simulink model "Practica_sincronica"  (R2021a)
settings: Solver=ode23tb  StartTime=0.0  StopTime=10  MaxStep=500e-6  RelTol=1e-4  EnableMultiTasking=on
libraries: fl_lib x2, spsRMSLib x2, spsThreePhaseVIMeasurementLib x2, nesl_utility x2, spsThreePhaseProgrammableVoltageSourceLib x1, spsThreePhaseSeriesRLCLoadLib x1, spsGroundLib x1, spsPowerLib x1, spsSynchronousMachinepuFundamentalLib x1, spsThreePhaseBreakerLib x1, spspowerguiLib x1
settings Model: ExtModeAutoUpdateStatusClock=off  Creator=MathWorks  LastModifiedBy=ontib
settings SolverCC: ZeroCrossAlgorithm=Adaptive  AlgebraicLoopSolver=TrustRegion
settings DataIOCC: LimitDataPoints=on  SaveFormat=Array  SignalLoggingSaveFormat=ModelDataLogs  ReturnWorkspaceOutputs=off
settings OptimizationCC: ExpressionDepthLimit=2147483647  InitFltsAndDblsToZero=on  EfficientMapNaN2IntZero=off  LifeSpan=inf
settings DebuggingCC: UnderspecifiedInitializationDetection=Classic  MergeDetectMultiDrivingBlocksExec=none  CheckExecutionContextPreStartOutputMsg=on  SignalResolutionControl=TryResolveAllWithWarning  SolverPrmCheckMsg=warning  MultiTaskDSMMsg=warning  MultiTaskCondExecSysMsg=none  SigSpecEnsureSampleTimeMsg=none  FcnCallInpInsideContextMsg=warning  StateNameClashWarn=warning  SFUnexpectedBacktrackingDiag=warning  SFNoUnconditionalDefaultTransitionDiag=warning  SFExecutionAtInitializationDiag=none  SFMachineParentedDataDiag=warning  ArithmeticOperatorsInVariantConditions=warning
settings HardwareCC: ProdBitPerPointer=32  ProdBitPerSizeT=32  ProdBitPerPtrDiffT=32  ProdLargestAtomicFloat=None  ProdIntDivRoundTo=Undefined  ProdEndianess=Unspecified  ProdWordSize=32  ProdHWDeviceType=32-bit Generic
settings ModelReferenceCC: PropagateSignalLabelsOutOfModel=off
settings SFSimCC: SimUseLocalCustomCode=off  CustomCodeUndefinedFunction=UseInterfaceOnly
settings RTWCC: RTWUseLocalCustomCode=off
settings CodeAppCC: StateflowObjectComments=on
settings GRTTargetCC: TargetFcnLib=ansi_tfl_tmw.mat  TargetLangStandard=C89/C90 (ANSI)  CombineOutputUpdateFcns=off  GRTInterface=on
settings ConfigComp: CovMetricSettings=dw  CovSaveCumulativeToWorkspaceVar=on  CovSaveSingleToWorkspaceVar=on  CovExternalEMLEnable=off  CovSFcnEnable=off
settings SimscapeCC: SimscapeNormalizeSystem=off

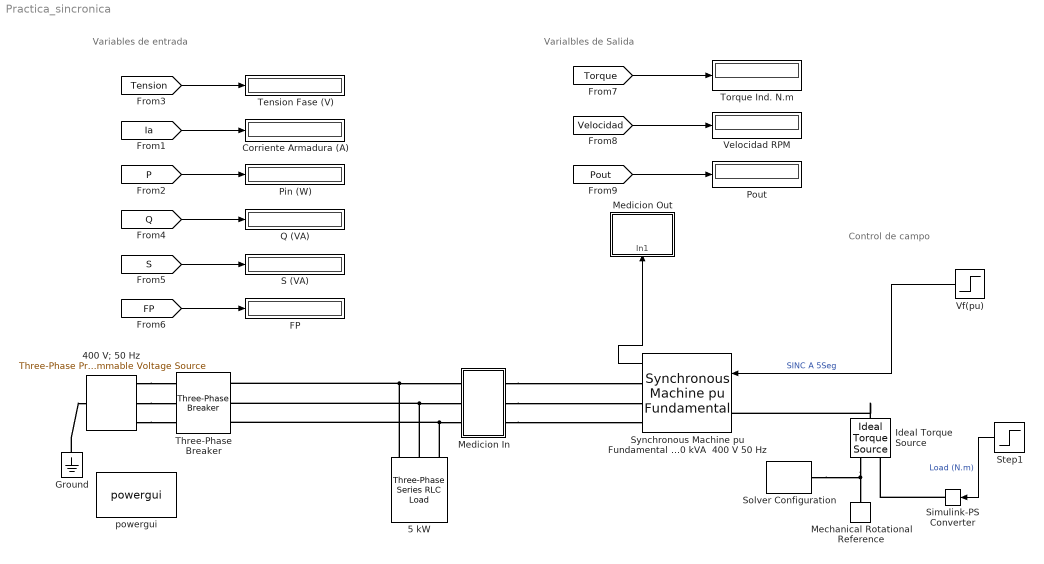
== system Practica_sincronica ==
  note: Varialbles de Salida
  note: Control de campo
  note: Variables de entrada
  400 V; 50 Hz : spsThreePhaseProgrammableVoltageSourceLib/Three-Phase Programmable Voltage Source  PositiveSequence="[400  0 50]"  VariationEntity=None  VariationType=Step  VariationTypeAlt=Step  VariationStep=0.5  VariationRate=10  VariationMagnitude=0.3  VariationFrequency=2  VariationTiming=[1 2]  VariationPhaseA=off  Amplitudes=[1 0.8 1.2 1.0]  TimeValues=[0 0.1 0.15 0.2]  HarmonicGeneration=off  HarmonicA=[3 0.2 -25 0]  HarmonicB=[2 0.15 35 2]  Timing="[0.05  3]"  BusType=swing  Pref=0  Qref=0  Qmin=-inf  Qmax=inf
  5 kW : spsThreePhaseSeriesRLCLoadLib/Three-Phase Series RLC Load  LConnTagsString=A|B|C  Configuration=Y (grounded)  NominalVoltage=400  Vabc=[1e3 1e3 1e3]  Vabcp=[1e3 1e3 1e3]  NominalFrequency=60  UnbalancedPower=off  ActivePower=5e3  InductivePower=0  CapacitivePower=0  Pabc=[10e3 9e3 11e3]  QLabc=[100 90 110]  QCabc=[100 90 110]  Pabcp=[10e3 9e3 11e3]  QLabcp=[100 90 110]  QCabcp=[100 90 110]  Measurements=None  LoadType=constant Z
  Corriente Armadura (A) : Display
      settings: Format=bank  Decimation=3
  FP : Display
  Ground : spsGroundLib/Ground  LConnTagsString=a
  Ideal Torque Source : fl_lib/Mechanical/Mechanical Sources/Ideal Torque Source
  Mechanical Rotational Reference : fl_lib/Mechanical/Rotational Elements/Mechanical Rotational Reference
  Medicion In : Subsystem
  Medicion Out : Subsystem
  Pin (W) : Display
      settings: Format=bank
  Pout : Display
      settings: Format=bank  Decimation=6
  Q (VA) : Display
      settings: Format=bank
  S (VA) : Display
      settings: Format=bank
  Simulink-PS Converter : nesl_utility/Simulink-PS Converter  PhysicalDomain=network_engine_domain  SubClassName=ps_input  LeftPortType=input  RightPortType=output  PseudoPeriodic=off  Frequencies=[]  NoiseDistribution=none  NoiseParameters=[]  Unit=1  AffineConversion=off  FilteringAndDerivatives=provide  SimscapeFilterOrder=1  InputFilterTimeConstant=0.001  UdotUserProvided=0
      settings: SourceProductBaseCode=PW,SS
  Solver Configuration : nesl_utility/Solver Configuration  PhysicalDomain=network_engine_domain  SubClassName=solver  LeftPortType=input  RightPortType=generic  Tones=[]  Harmonics=[]  SimulateNoise=off  Profile=off  UseLocalSampling=off  EnableSwitchedLinearOptims=on  FrequencyDomain=off  UseCCode=off  RelTol=0.001  AbsTol=1e-06  MinStep=1e-09  ToWorkspace=off  RevertToSquareIcSolve=off  NumHomotopyIterations=100  PhasorMode=off  PhasorModeNumHarmonics=1  DoDC=off  ResidualTolerance=1e-09  UseLocalSolver=off  LocalSolverChoice=NE_BACKWARD_EULER_ADVANCER  LocalSolverSampleTime=0.001  DoFixedCost=off  MaxNonlinIter=3  MaxModeIter=2  ComputeImpulses=off  ImpulseIterations=2  LinearAlgebra=auto  EquationFormulation=NE_TIME_EF  DelaysMemoryBudget=1024  AutomaticFiltering=on  FilteringTimeConstant=0.001  PartitionStorageMethod=AS_NEEDED  PartitionMemoryBudget=1024  PartitionMethod=ROBUST
      settings: SourceProductBaseCode=PW,SS
  Step1 : Step  Time=6  After=280  SampleTime=0
  Synchronous Machine pu Fundamental 60 kVA  400 V 50 Hz : spsSynchronousMachinepuFundamentalLib/Synchronous Machine pu Fundamental  PresetModel=No  MechanicalLoad=Mechanical rotational port  ShowDetailedParameters=on  RotorType=Round  Units=per unit fundamental parameters  MeasurementBus=off  NominalParameters=[6e+004 400 50]  Stator=[0.03788 0.08 2.16 0.94]  Field=[0.02124 0.1719]  Dampers2=[0.0652, 0.5134, 0.0287, 0.2553, 7.765e-3, 0.9167 ]  Dampers1=[0.1463 0.3085 0.05754 0.05281]  Mechanical=[1.0 0.02056 2]  PolePairs=2  InitialConditions="[ -100  0  0  0  0  0  0  0  1 ]"  SetSaturation=off  Saturation=[0.6404,0.7127,0.8441,0.9214,0.9956,1.082,1.19,1.316,1.457;0.7,0.7698,0.8872,0.9466,0.9969,1.046,1.1,1.151,1.201]  LoadFlowParameters=[1,0,0,0,0]  TsPowergui=0  TsBlock=-1  IterativeModel=Trapezoidal non iterative  IterativeDiscreteModel=Trapezoidal non iterative  BusType=PV  Pref=0  Qref=0  Qmin=-inf  Qmax=inf  PLF=0  QLF=0
      settings: SourceProductBaseCode=PS
  Tension Fase (V) : Display
      settings: Format=bank  Decimation=3
  Three-Phase Breaker : spsThreePhaseBreakerLib/Three-Phase Breaker  InitialState=open  SwitchA=on  SwitchB=on  SwitchC=on  SwitchTimes=[0.01]  External=off  BreakerResistance=0.001  SnubberResistance=1e5  SnubberCapacitance=inf  Measurements=None
  Torque Ind. N.m : Display
  Velocidad RPM : Display
      settings: Decimation=6
  Vf(pu) : Step  Time=5  After=1.6  SampleTime=0
  powergui : spspowerguiLib/powergui  Priority=2  SimulationMode=Continuous  SampleTime=0  frequency=50  Iterations=50  frequencyindice=50  Pbase=100e6  ErrMax=1e-4  UnitsV=kV  UnitsW=MW  buscounter=0  FunctionMessages=off  echomessages=off  EnableUseOfTLC=off  CurrentSourceSwitches=off  DisableSnubberDevices=off  DisableRonSwitches=off  DisableVfSwitches=off  DisplayEquations=off  AutomaticDiscreteSolvers=off  SolverType=Tustin  Interpol=off  ExternalGateDelay=off  methode=off  Ts=0  x0status=blocks  SPID=on  SwTol=0  HookPort=off  NonlinearTolerance=1e-4  nMaxIteration=100  ContinueOnMaxIteration=off  RestoreLinks=warning  ResistiveCurrentMeasurement=off  Frange=[0:2:500]  Ylog=off  Xlog=on  ShowGrid=off  save=off  variable=ZData  structure=0  ZoomFFT=on  StartTime=0.0  cycles=1  DisplayStyle=1  fundamental=60  FreqAxis=off  MaxFrequency=1000  frequencyindicesteady=1  RmsSteady=1  display=off
  wires:
  Vf(pu)/1 -> Synchronous Machine pu Fundamental 60 kVA  400 V 50 Hz/1  "SINC A 5Seg"
  Step1/1 -> Simulink-PS Converter/1  "Load (N.m)"
  [Tension] -> Tension Fase (V)/1
  [Ia] -> Corriente Armadura (A)/1
  [Q] -> Q (VA)/1
  [P] -> Pin (W)/1
  [S] -> S (VA)/1
  [FP] -> FP/1
  Synchronous Machine pu Fundamental 60 kVA  400 V 50 Hz/1 -> Medicion Out/1(In1)
  [Pout] -> Pout/1
  [Velocidad] -> Velocidad RPM/1
  [Torque] -> Torque Ind. N.m/1
  connections:
  400 V; 50 Hz/RConn1 -- Three-Phase Breaker/LConn1
  400 V; 50 Hz/RConn2 -- Three-Phase Breaker/LConn2
  400 V; 50 Hz/RConn3 -- Three-Phase Breaker/LConn3
  Ground/LConn1 -- 400 V; 50 Hz/LConn1
  5 kW/LConn1 -- Three-Phase Breaker/RConn1 -- Medicion In/LConn1
  5 kW/LConn2 -- Three-Phase Breaker/RConn2 -- Medicion In/LConn2
  5 kW/LConn3 -- Three-Phase Breaker/RConn3 -- Medicion In/LConn3
  Medicion In/RConn1 -- Synchronous Machine pu Fundamental 60 kVA  400 V 50 Hz/RConn1
  Medicion In/RConn2 -- Synchronous Machine pu Fundamental 60 kVA  400 V 50 Hz/RConn2
  Medicion In/RConn3 -- Synchronous Machine pu Fundamental 60 kVA  400 V 50 Hz/RConn3
  Solver Configuration/RConn1 -- Mechanical Rotational Reference/LConn1 -- Ideal Torque Source/RConn2
  Ideal Torque Source/LConn1 -- Synchronous Machine pu Fundamental 60 kVA  400 V 50 Hz/LConn1
  Simulink-PS Converter/RConn1 -- Ideal Torque Source/RConn1

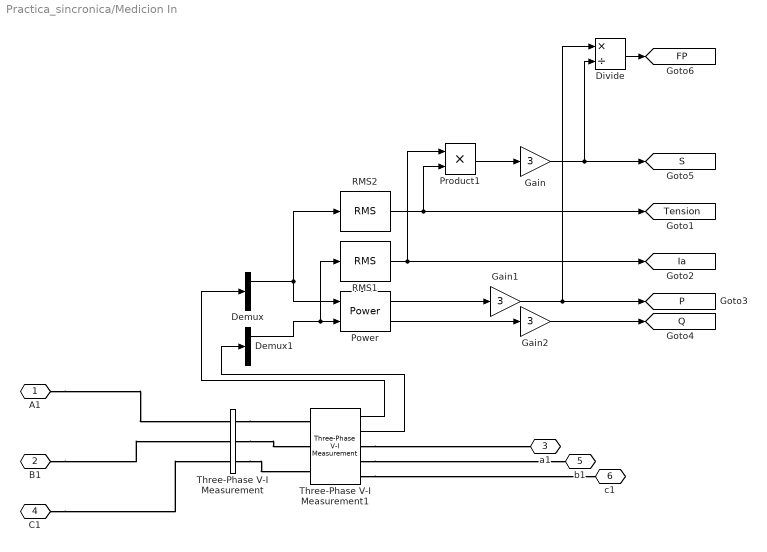
== system Practica_sincronica/Medicion In ==
  Demux : Demux  Outputs=3
  Demux1 : Demux  Outputs=3
  Divide : Product  Inputs=*/
  Gain : Gain  Gain=3
  Gain1 : Gain  Gain=3
  Gain2 : Gain  Gain=3
  Power : spsPowerLib/Power  Freq=50  Vinit=[1, 0]  Iinit=[1, 0]  Ts=0
      settings: SourceProductBaseCode=PS
  Product1 : Product
  RMS1 : spsRMSLib/RMS  TrueRMS=off  Freq=50  RMSInit=0  Ts=0
  RMS2 : spsRMSLib/RMS  TrueRMS=off  Freq=50  RMSInit=0  Ts=0
  Three-Phase V-I Measurement : spsThreePhaseVIMeasurementLib/Three-Phase V-I Measurement  VoltageMeasurement=phase-to-ground  SetLabelV=on  LabelV=Vabc  Vpu=off  VpuLL=off  CurrentMeasurement=no  SetLabelI=off  LabelI=Iabc  Ipu=off  Pbase=100e6  Vbase=500e3  OutputType=Complex  PhasorSimulation=off  PSBequivalent=0
  Three-Phase V-I Measurement1 : spsThreePhaseVIMeasurementLib/Three-Phase V-I Measurement  VoltageMeasurement=phase-to-ground  SetLabelV=off  LabelV=Vabc  Vpu=off  VpuLL=off  CurrentMeasurement=yes  SetLabelI=off  LabelI=Iabc  Ipu=off  Pbase=100e6  Vbase=500e3  OutputType=Complex  PhasorSimulation=off  PSBequivalent=0
  A1 : PMIOPort  Side=Left
  B1 : PMIOPort  Port=2  Side=Left
  a1 : PMIOPort  Port=3  Side=Right
  C1 : PMIOPort  Port=4  Side=Left
  b1 : PMIOPort  Port=5  Side=Right
  c1 : PMIOPort  Port=6  Side=Right
  tag scope: FP=global, Ia=global, P=global, Q=global, S=global, Tension=global
  wires:
  Gain2/1 -> [Q]
  Gain1/1 -> Divide/1, [P]
  RMS1/1 -> [Ia], Product1/1
  Power/2 -> Gain2/1
  Three-Phase V-I Measurement1/2 -> Demux1/1
  Three-Phase V-I Measurement1/1 -> Demux/1
  Demux/1 -> Power/1, RMS2/1
  RMS2/1 -> [Tension], Product1/2
  Product1/1 -> Gain/1
  Power/1 -> Gain1/1
  Demux1/1 -> RMS1/1, Power/2
  Gain/1 -> Divide/2, [S]
  Divide/1 -> [FP]
  connections:
  B1/RConn1 -- Three-Phase V-I Measurement/LConn2
  Three-Phase V-I Measurement/RConn2 -- Three-Phase V-I Measurement1/LConn2
  C1/RConn1 -- Three-Phase V-I Measurement/LConn3
  Three-Phase V-I Measurement1/RConn3 -- c1/RConn1
  Three-Phase V-I Measurement1/RConn2 -- b1/RConn1
  A1/RConn1 -- Three-Phase V-I Measurement/LConn1
  Three-Phase V-I Measurement/RConn1 -- Three-Phase V-I Measurement1/LConn1
  Three-Phase V-I Measurement/RConn3 -- Three-Phase V-I Measurement1/LConn3
  Three-Phase V-I Measurement1/RConn1 -- a1/RConn1

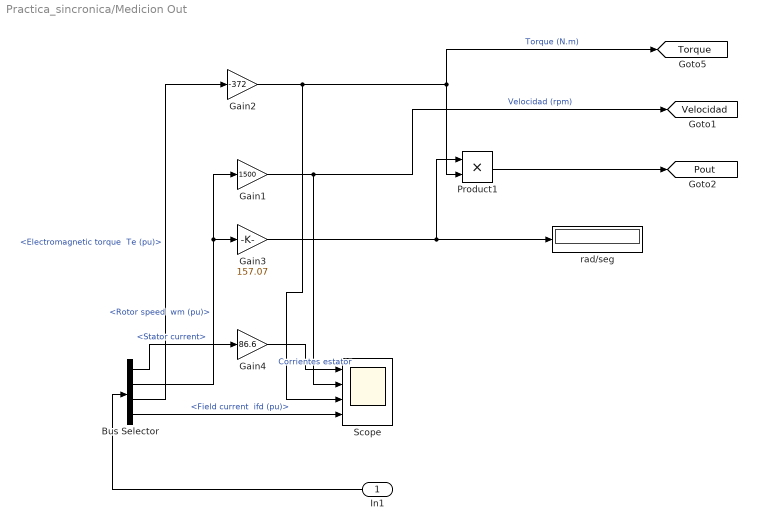
== system Practica_sincronica/Medicion Out ==
  In1 : Inport
  Bus Selector : BusSelector  OutputSignals="Stator current,Mechanical.Rotor speed  wm (pu),Mechanical.Electromagnetic torque  Te (pu),dq0 components.Field current  ifd (pu)"
  Gain1 : Gain  Gain=1500
  Gain2 : Gain  Gain=-372
  Gain3 : Gain  Gain=157.07
  Gain4 : Gain  Gain=86.6
  Product1 : Product
  Scope : Scope  NumInputPorts=4
  rad/seg : Display
      settings: Decimation=6
  tag scope: Pout=global, Torque=global, Velocidad=global
  wires:
  Bus Selector/1 -> Gain4/1  "<Stator current>"
  Product1/1 -> [Pout]
  Bus Selector/4 -> Scope/4  "<Field current  ifd (pu)>"
  In1/1 -> Bus Selector/1
  Gain4/1 -> Scope/1  "Corrientes estator"
  Bus Selector/2 -> Gain1/1, Gain3/1  "<Rotor speed  wm (pu)>"
  Gain3/1 -> rad/seg/1, Product1/1
  Bus Selector/3 -> Gain2/1  "<Electromagnetic torque  Te (pu)>"
  Gain1/1 -> Scope/2, [Velocidad]  "Velocidad (rpm)"
  Gain2/1 -> Scope/3, [Torque], Product1/2  "Torque (N.m)"
